simulink model "Superposition"  (R2020a)
settings: Solver=VariableStepAuto  StartTime=0.0  StopTime=0.50  RelTol=1e-3
libraries: powerlib x16, powerlib_meascontrol x6
settings Model: Creator=Alisamar  LastModifiedBy=Alisamar

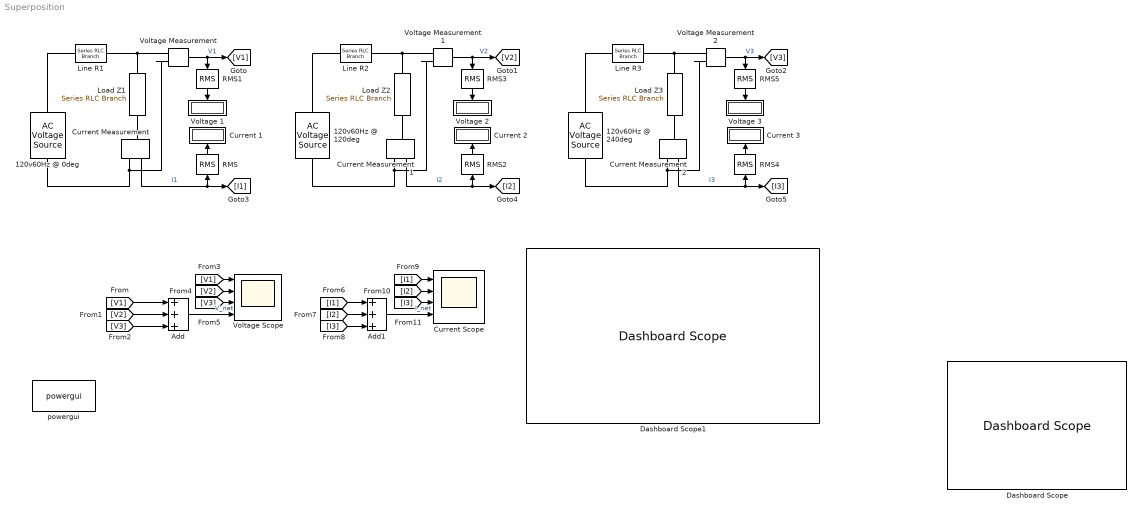
== system Superposition ==
  120v60Hz @ 0deg : powerlib/Electrical Sources/AC Voltage Source  Amplitude=120  Phase=0  Frequency=60  SampleTime=0  Measurements=None  BusType=swing  Pref=10e3  Qref=0  Qmin=-inf  Qmax=+inf
  120v60Hz @ 120deg : powerlib/Electrical Sources/AC Voltage Source  Amplitude=120  Phase=120  Frequency=60  SampleTime=0  Measurements=None  BusType=swing  Pref=10e3  Qref=0  Qmin=-inf  Qmax=+inf
  120v60Hz @ 240deg : powerlib/Electrical Sources/AC Voltage Source  Amplitude=120  Phase=240  Frequency=60  SampleTime=0  Measurements=None  BusType=swing  Pref=10e3  Qref=0  Qmin=-inf  Qmax=+inf
  Add : Sum  Inputs=+++
  Add1 : Sum  Inputs=+++
  Current Scope : Scope  NumInputPorts=4
  Current 1 : Display
  Current 2 : Display
  Current 3 : Display
  Current Measurement : powerlib/Measurements/Current Measurement  PhasorSimulation=off  OutputType=Complex  PSBequivalent=0
  Current Measurement1 : powerlib/Measurements/Current Measurement  PhasorSimulation=off  OutputType=Complex  PSBequivalent=0
  Current Measurement2 : powerlib/Measurements/Current Measurement  PhasorSimulation=off  OutputType=Complex  PSBequivalent=0
  Dashboard Scope : DashboardScope
  Dashboard Scope1 : DashboardScope
  Line R1 : powerlib/Elements/Series RLC Branch  LConnTagsString=__new0  RConnTagsString=__new0  BranchType=R  Resistance=5  Inductance=0  SetiL0=off  InitialCurrent=0  Capacitance=0  Setx0=off  InitialVoltage=0  Measurements=None
  Line R2 : powerlib/Elements/Series RLC Branch  LConnTagsString=__new0  RConnTagsString=__new0  BranchType=R  Resistance=5  Inductance=0  SetiL0=off  InitialCurrent=0  Capacitance=0  Setx0=off  InitialVoltage=0  Measurements=None
  Line R3 : powerlib/Elements/Series RLC Branch  LConnTagsString=__new0  RConnTagsString=__new0  BranchType=R  Resistance=5  Inductance=0  SetiL0=off  InitialCurrent=0  Capacitance=0  Setx0=off  InitialVoltage=0  Measurements=None
  Load Z1 : powerlib/Elements/Series RLC Branch  LConnTagsString=__new0  RConnTagsString=__new0  BranchType=RLC  Resistance=100  Inductance=0.0025  SetiL0=off  InitialCurrent=0  Capacitance=0.000001  Setx0=off  InitialVoltage=0  Measurements=None
  Load Z2 : powerlib/Elements/Series RLC Branch  LConnTagsString=__new0  RConnTagsString=__new0  BranchType=RLC  Resistance=100  Inductance=0.0025  SetiL0=off  InitialCurrent=0  Capacitance=0.000001  Setx0=off  InitialVoltage=0  Measurements=None
  Load Z3 : powerlib/Elements/Series RLC Branch  LConnTagsString=__new0  RConnTagsString=__new0  BranchType=RLC  Resistance=100  Inductance=0.0025  SetiL0=off  InitialCurrent=0  Capacitance=0.000001  Setx0=off  InitialVoltage=0  Measurements=None
  RMS{,1..5} (6 alike) : powerlib_meascontrol/Measurements/RMS  TrueRMS=on  Freq=60  RMSInit=120  Ts=0
  Voltage Scope : Scope  NumInputPorts=4
  Voltage 1 : Display
  Voltage 2 : Display
  Voltage 3 : Display
  Voltage Measurement : powerlib/Measurements/Voltage Measurement  PhasorSimulation=off  OutputType=Complex  PSBequivalent=0
  Voltage Measurement1 : powerlib/Measurements/Voltage Measurement  PhasorSimulation=off  OutputType=Complex  PSBequivalent=0
  Voltage Measurement2 : powerlib/Measurements/Voltage Measurement  PhasorSimulation=off  OutputType=Complex  PSBequivalent=0
  powergui : powerlib/powergui  Priority=1  SimulationMode=Continuous  SampleTime=50e-6  frequency=60  Iterations=50  frequencyindice=60  Pbase=100e6  ErrMax=1e-4  UnitsV=kV  UnitsW=MW  buscounter=0  FunctionMessages=off  echomessages=off  EnableUseOfTLC=off  CurrentSourceSwitches=off  DisableSnubberDevices=off  DisableRonSwitches=off  DisableVfSwitches=off  DisplayEquations=off  AutomaticDiscreteSolvers=off  SolverType=Tustin/Backward Euler (TBE)  Interpol=off  ExternalGateDelay=off  methode=off  Ts=100  x0status=blocks  SPID=on  SwTol=0  HookPort=off  NonlinearTolerance=1e-4  nMaxIteration=100  ContinueOnMaxIteration=off  RestoreLinks=warning  ResistiveCurrentMeasurement=off  Frange=[0:2:500]  Ylog=off  Xlog=on  ShowGrid=off  save=off  variable=ZData  structure=0  ZoomFFT=off  StartTime=0.0  cycles=1  DisplayStyle=1  fundamental=60  FreqAxis=off  MaxFrequency=1000  frequencyindicesteady=1  RmsSteady=1  display=off
  wires:
  RMS/1 -> Current 1/1
  Current Measurement/1 -> [I1], RMS/1  "I1"
  Voltage Measurement/1 -> [V1], RMS1/1  "V1"
  Voltage Measurement1/1 -> [V2], RMS3/1  "V2"
  Current Measurement1/1 -> [I2], RMS2/1  "I2"
  RMS3/1 -> Voltage 2/1
  RMS2/1 -> Current 2/1
  Voltage Measurement2/1 -> [V3], RMS5/1  "V3"
  RMS5/1 -> Voltage 3/1
  RMS4/1 -> Current 3/1
  Current Measurement2/1 -> [I3], RMS4/1  "I3"
  Add/1 -> Voltage Scope/4  "V_net"
  Add1/1 -> Current Scope/4  "I_net"
  RMS1/1 -> Voltage 1/1
  [V2] -> Add/2
  [V1] -> Add/1
  [V3] -> Add/3
  [V1] -> Voltage Scope/1
  [V2] -> Voltage Scope/2
  [V3] -> Voltage Scope/3
  [I2] -> Add1/2
  [I2] -> Current Scope/2
  [I1] -> Add1/1
  [I3] -> Add1/3
  [I1] -> Current Scope/1
  [I3] -> Current Scope/3
  connections:
  120v60Hz @ 0deg/RConn1 -- Line R1/LConn1
  Load Z1/LConn1 -- Line R1/RConn1 -- Voltage Measurement/LConn1
  120v60Hz @ 0deg/LConn1 -- Voltage Measurement/LConn2 -- Current Measurement/RConn1
  Load Z1/RConn1 -- Current Measurement/LConn1
  Load Z2/LConn1 -- Line R2/RConn1 -- Voltage Measurement1/LConn1
  Current Measurement1/RConn1 -- 120v60Hz @ 120deg/LConn1 -- Voltage Measurement1/LConn2
  Load Z2/RConn1 -- Current Measurement1/LConn1
  120v60Hz @ 120deg/RConn1 -- Line R2/LConn1
  Current Measurement2/RConn1 -- 120v60Hz @ 240deg/LConn1 -- Voltage Measurement2/LConn2
  Load Z3/LConn1 -- Line R3/RConn1 -- Voltage Measurement2/LConn1
  Load Z3/RConn1 -- Current Measurement2/LConn1
  120v60Hz @ 240deg/RConn1 -- Line R3/LConn1
